simulink model "Force_calc"  (R2020b)
settings: Solver=VariableStepAuto  StartTime=0.0  StopTime=10.0  RelTol=1e-3
undefined symbols (not defined in the file): CTgain
libraries: fl_lib x28, sm_lib x4
settings Model: Creator=jbmic  LastModifiedBy=jbmic

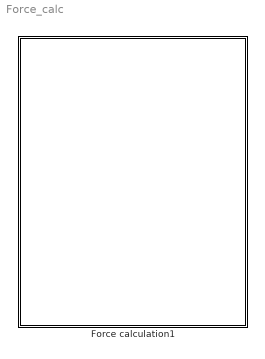
== system Force_calc ==
  Force calculation1 : Subsystem

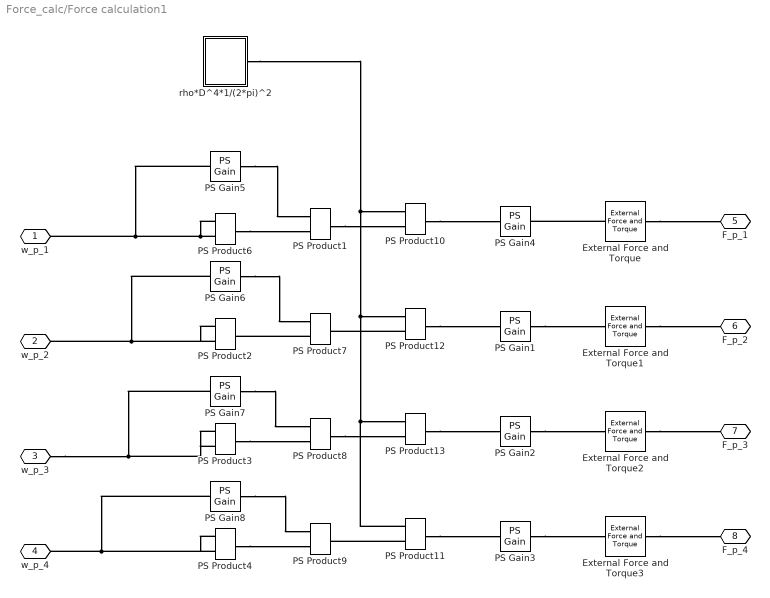
== system Force_calc/Force calculation1 ==
  External Force and Torque{,1..3} (4 alike) : sm_lib/Forces and Torques/External Force and Torque  ForceResolutionFrame=AttachedFrame  EnableForceX=off  EnableForceY=off  EnableForceZ=on  EnableForce=off  TorqueResolutionFrame=AttachedFrame  EnableTorqueX=off  EnableTorqueY=off  EnableTorqueZ=off  EnableTorque=off
  PS Gain1 : fl_lib/Physical Signals/Functions/PS Gain  gain=1
  PS Gain2 : fl_lib/Physical Signals/Functions/PS Gain  gain=-1
  PS Gain3 : fl_lib/Physical Signals/Functions/PS Gain  gain=-1
  PS Gain4 : fl_lib/Physical Signals/Functions/PS Gain  gain=1
  PS Gain{5..8} (4 alike) : fl_lib/Physical Signals/Functions/PS Gain  gain=CTgain 1/(rad/s)
  PS Product{1..4,6..13} (12 alike) : fl_lib/Physical Signals/Functions/PS Product
  rho*D^4*1/(2*pi)^2 : Subsystem
  w_p_1 : PMIOPort  Side=Left
  w_p_2 : PMIOPort  Port=2  Side=Left
  w_p_3 : PMIOPort  Port=3  Side=Left
  w_p_4 : PMIOPort  Port=4  Side=Left
  F_p_1 : PMIOPort  Port=5  Side=Left
  F_p_2 : PMIOPort  Port=6  Side=Left
  F_p_3 : PMIOPort  Port=7  Side=Left
  F_p_4 : PMIOPort  Port=8  Side=Left
  connections:
  External Force and Torque2/RConn1 -- F_p_3/RConn1
  External Force and Torque/RConn1 -- F_p_1/RConn1
  External Force and Torque1/RConn1 -- F_p_2/RConn1
  External Force and Torque3/RConn1 -- F_p_4/RConn1
  PS Product6/LConn2 -- PS Product6/LConn1 -- w_p_1/RConn1 -- PS Gain5/LConn1
  PS Product11/LConn2 -- PS Product9/RConn1
  PS Product12/LConn2 -- PS Product7/RConn1
  PS Product8/RConn1 -- PS Product13/LConn2
  rho*D^4*1/(2*pi)^2/RConn1 -- PS Product12/LConn1 -- PS Product11/LConn1 -- PS Product13/LConn1 -- PS Product10/LConn1
  External Force and Torque/LConn1 -- PS Gain4/RConn1
  PS Gain1/RConn1 -- External Force and Torque1/LConn1
  PS Gain2/RConn1 -- External Force and Torque2/LConn1
  PS Gain3/RConn1 -- External Force and Torque3/LConn1
  PS Product10/RConn1 -- PS Gain4/LConn1
  PS Product12/RConn1 -- PS Gain1/LConn1
  PS Product13/RConn1 -- PS Gain2/LConn1
  PS Product11/RConn1 -- PS Gain3/LConn1
  PS Product6/RConn1 -- PS Product1/LConn2
  PS Product1/RConn1 -- PS Product10/LConn2
  PS Gain5/RConn1 -- PS Product1/LConn1
  PS Gain6/LConn1 -- w_p_2/RConn1 -- PS Product2/LConn2 -- PS Product2/LConn1
  PS Gain6/RConn1 -- PS Product7/LConn1
  PS Product7/LConn2 -- PS Product2/RConn1
  PS Gain7/LConn1 -- w_p_3/RConn1 -- PS Product3/LConn2 -- PS Product3/LConn1
  PS Gain7/RConn1 -- PS Product8/LConn1
  PS Product3/RConn1 -- PS Product8/LConn2
  PS Gain8/LConn1 -- w_p_4/RConn1 -- PS Product4/LConn2 -- PS Product4/LConn1
  PS Gain8/RConn1 -- PS Product9/LConn1
  PS Product4/RConn1 -- PS Product9/LConn2

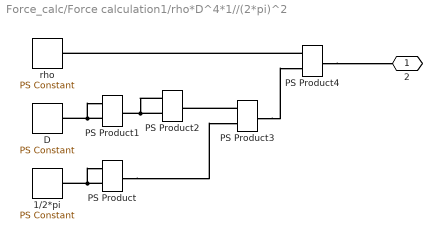
== system Force_calc/Force calculation1/rho*D^4*1//(2*pi)^2 ==
  1/2*pi : fl_lib/Physical Signals/Sources/PS Constant  constant=1/(2*pi) 1/rad
  D : fl_lib/Physical Signals/Sources/PS Constant  constant=0.1016 m
  PS Product{,1..4} (5 alike) : fl_lib/Physical Signals/Functions/PS Product
  rho : fl_lib/Physical Signals/Sources/PS Constant  constant=1.225 kg/m^3
  2 : PMIOPort  Side=Right
  connections:
  PS Product3/RConn1 -- PS Product4/LConn2
  PS Product/RConn1 -- PS Product3/LConn2
  PS Product4/RConn1 -- 2/RConn1
  PS Product2/LConn2 -- PS Product2/LConn1 -- PS Product1/RConn1
  PS Product1/LConn2 -- PS Product1/LConn1 -- D/RConn1
  PS Product/LConn2 -- PS Product/LConn1 -- 1/2*pi/RConn1
  PS Product4/LConn1 -- rho/RConn1
  PS Product3/LConn1 -- PS Product2/RConn1
